simulink model "EarlyReturn12_2018a"  (R2018a)
settings: Solver=VariableStepAuto  StartTime=0.0  StopTime=0.1  RelTol=1e-3
settings Model: Creator=BEAR  LastModifiedBy=bzhan

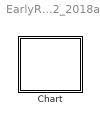
== system EarlyReturn12_2018a ==
  Chart : Stateflow chart  TreatAsAtomicUnit=on

== stateflow chart EarlyReturn12_2018a/Chart ==
  state A
    en: E;f("enA_done")
  state B
    en: f("enB")
  state C
    en: f("enC")
  (default) -> A
  A -> B : E
  B -> C
  data: s function_input
  events: E local FUNCTION_CALL_EVENT
  function f(s):
    | function f(s)
    |   fprintf(s+"\n");
